simulink model "population_growth"  (R2017b)
settings: Solver=FixedStepDiscrete  StartTime=2010  StopTime=2100  FixedStep=1  MaxStep=1  RelTol=1e-3  EnableMultiTasking=on
PostLoadFcn:
  | load model_parameters
  | % msgbox('Model parameters loaded into base workspace!','Loaded')
values from neighbouring files (symbols this model uses):
  P_2010 = round([P_2010 P_2010].*[male_ratio(1:101) (1-male_ratio(1:101))])    [define_data.m]    (also in model_parameters.mat = [2183279 2225429 2206265 2148270 2142055 2136850 2109005 211)
  p_death_f = ATable(:,5)    [define_data.m]    (also in model_parameters.mat = [0.006096 0.000434 0.000256 0.000192 0.000148 0.000136 0.000)
  p_death_m = ATable(:,2)    [define_data.m]    (also in model_parameters.mat = [0.007379 0.000494 0.000317 0.000241 0.0002 0.000179 0.00016)
  P_immigrants = round(P_immigrants)    [define_data.m]    (also in model_parameters.mat = [0 0 0 0 0 0 0 0 0 0 0 0 ... (240 elements, 120x2)])
  r_birth = [zeros(10,1) ... (first row only)    [define_data.m]    (also in model_parameters.mat = [0 0 0 0 0 0 0 0 0 0 0.4 0.4 ... (120 elements, 120x1)])
libraries: simulink x1
Description:
  | This model predicts the population of the
  | United States as it evolves over the next
  | century. Population for the year 2010 and
  | birth rates were gathered from the US
  | Census Bureau. Immigration rates were
  | derived from DHS, and death rates were
  | provided by the Social Security
  | Administration. These parameters are held
  | fixed and propagated forward.
settings Model: Creator=wcampbel  LastModifiedBy=wcampbel
settings DataIOCC: LimitDataPoints=on  SaveFormat=Array
settings OptimizationCC: ExpressionDepthLimit=2147483647  LifeSpan=inf
settings DebuggingCC: SolverPrmCheckMsg=warning  StateNameClashWarn=warning  SFUnexpectedBacktrackingDiag=warning  SFNoUnconditionalDefaultTransitionDiag=warning  SFExecutionAtInitializationDiag=none
settings HardwareCC: ProdBitPerPointer=32  ProdBitPerSizeT=32  ProdBitPerPtrDiffT=32  ProdLargestAtomicFloat=None  ProdIntDivRoundTo=Undefined  ProdEndianess=Unspecified  ProdWordSize=32  ProdHWDeviceType=32-bit Generic
settings ModelReferenceCC: PropagateSignalLabelsOutOfModel=off
settings CodeAppCC: StateflowObjectComments=on
settings GRTTargetCC: TargetLangStandard=C89/C90 (ANSI)  GeneratePreprocessorConditionals=Disable all  CombineOutputUpdateFcns=off  GRTInterface=on
settings ConfigComp: CovMetricSettings=dw  CovHtmlReporting=on  CovSaveCumulativeToWorkspaceVar=on  CovSaveSingleToWorkspaceVar=on  CovExternalEMLEnable=off

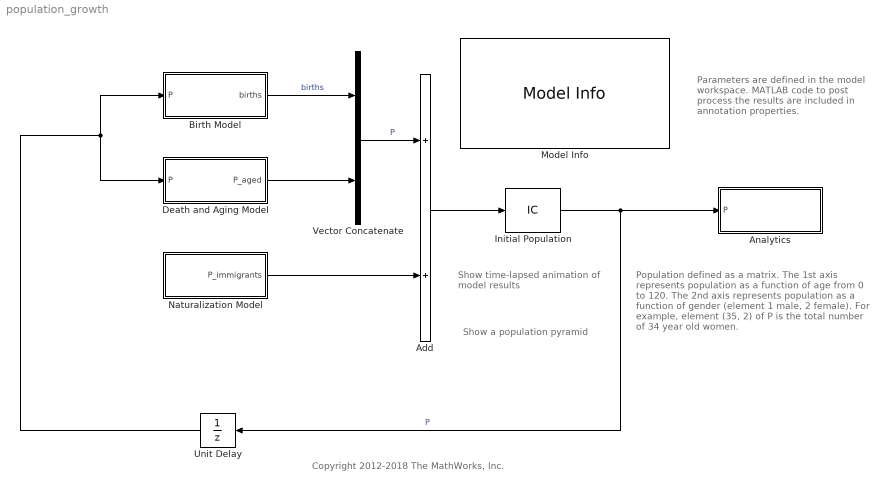
== system population_growth ==
  note: Population defined as a matrix.
      |
      | The 1st axis represents population as
      | a function of age from 0 to 120.
      |
      | The 2nd axis represents population as
      | a function of gender (element 1 male,
      | 2 female).
      |
      | For example, element (35, 2) of P is the
      | total number of 34 year old women.
  note: Parameters are defined in the
      | model workspace. MATLAB code
      | to post process the results are
      | included in annotation properties.
  note: Show a population pyramid
  note: Show time-lapsed animation
      | of model results
  note: Copyright 2012-2018 The MathWorks, Inc.
  Add : Sum
  Analytics : Subsystem
  Birth Model : Subsystem
  Death and Aging Model : Subsystem
  Initial Population : InitialCondition  Priority=3000  Value=P_2010
  Model Info : simulink/Model-Wide Utilities/Model Info  Frame=on  DisplayStringWithTags=%<Description>  HorizontalTextAlignment=Left  LeftAlignmentValue=0.02
  Naturalization Model : Subsystem
  Unit Delay : UnitDelay  SampleTime=-1
  Vector Concatenate : Concatenate  Mode=Multidimensional array
  wires:
  Birth Model/1(births) -> Vector Concatenate/1  "births"
  Death and Aging Model/1(P_aged) -> Vector Concatenate/2
  Naturalization Model/1(P_immigrants) -> Add/2
  Vector Concatenate/1 -> Add/1  "P"
  Add/1 -> Initial Population/1
  Unit Delay/1 -> Birth Model/1(P), Death and Aging Model/1(P)
  Initial Population/1 -> Analytics/1(P), Unit Delay/1  "P"

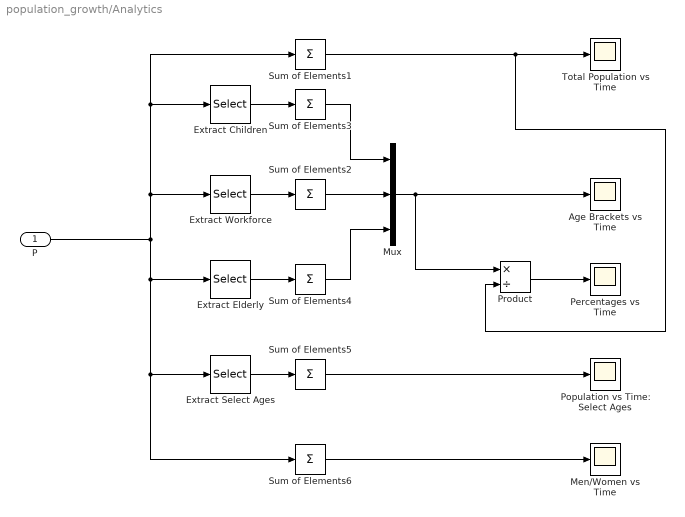
== system population_growth/Analytics ==
  P : Inport
  Age Brackets vs Time : Scope
      settings: Priority=1
  Extract Children : Selector  NumberOfDimensions=2  InputPortWidth=3  IndexOptions=Index vector (dialog),Select all  Indices=[1:18],2  OutputSizes=1,1
  Extract Elderly : Selector  NumberOfDimensions=2  InputPortWidth=3  IndexOptions=Index vector (dialog),Select all  Indices=[67:120],2  OutputSizes=1,1
  Extract Select Ages : Selector  NumberOfDimensions=2  InputPortWidth=3  IndexOptions=Index vector (dialog),Select all  Indices=[1:10:120],2  OutputSizes=1,1
  Extract Workforce : Selector  NumberOfDimensions=2  InputPortWidth=3  IndexOptions=Index vector (dialog),Select all  Indices=[19:66],2  OutputSizes=1,1
  Men/Women vs Time : Scope
      settings: Priority=1
  Mux : Mux  Inputs=3
  Percentages vs Time : Scope
      settings: Priority=1
  Population vs Time: Select Ages : Scope
      settings: Priority=1
  Product : Product  Inputs=*/  RndMeth=Zero
  Sum of Elements{1..4} (4 alike) : Sum  Inputs=+  CollapseDim=2
  Sum of Elements5 : Sum  Inputs=+  CollapseMode=Specified dimension  CollapseDim=2
  Sum of Elements6 : Sum  Inputs=+  CollapseMode=Specified dimension
  Total Population vs Time : Scope
      settings: Priority=1
  wires:
  Sum of Elements1/1 -> Total Population vs Time/1, Product/2
  P/1 -> Sum of Elements1/1, Extract Children/1, Extract Workforce/1, Extract Select Ages/1, Sum of Elements6/1, Extract Elderly/1
  Extract Workforce/1 -> Sum of Elements2/1
  Sum of Elements2/1 -> Mux/2
  Extract Children/1 -> Sum of Elements3/1
  Extract Elderly/1 -> Sum of Elements4/1
  Mux/1 -> Age Brackets vs Time/1, Product/1
  Sum of Elements3/1 -> Mux/1
  Sum of Elements4/1 -> Mux/3
  Product/1 -> Percentages vs Time/1
  Extract Select Ages/1 -> Sum of Elements5/1
  Sum of Elements5/1 -> Population vs Time: Select Ages/1
  Sum of Elements6/1 -> Men/Women vs Time/1

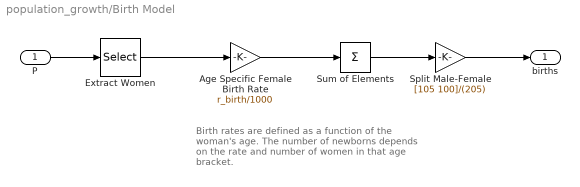
== system population_growth/Birth Model ==
  note: Birth rates are defined as a function
      | of the woman's age. The number of
      | newborns depends on the rate and
      | number of women in that age bracket.
  P : Inport
  Age Specific Female Birth Rate : Gain  Gain=r_birth/1000
  Extract Women : Selector  NumberOfDimensions=2  InputPortWidth=3  IndexOptions=Select all,Index vector (dialog)  Indices=[1 3],2  OutputSizes=1,1
  Split Male-Female : Gain  Gain=[105 100]/(205)
  Sum of Elements : Sum  Inputs=+
  births : Outport
  wires:
  P/1 -> Extract Women/1
  Age Specific Female Birth Rate/1 -> Sum of Elements/1
  Sum of Elements/1 -> Split Male-Female/1
  Extract Women/1 -> Age Specific Female Birth Rate/1
  Split Male-Female/1 -> births/1

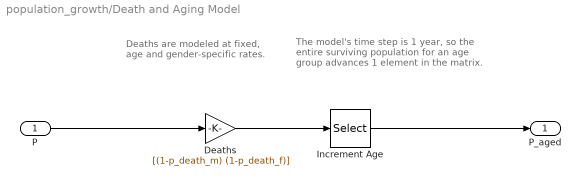
== system population_growth/Death and Aging Model ==
  note: Deaths are modeled
      | at fixed, age and
      | gender-specific rates.
  note: The model's time step is 1 year,
      | so the entire surviving population
      | for an age group advances 1
      | element in the matrix.
  P : Inport
  Deaths : Gain  Gain=[(1-p_death_m) (1-p_death_f)]
  Increment Age : Selector  NumberOfDimensions=2  InputPortWidth=101  IndexOptions=Index vector (dialog),Select all  Indices=[1:119],1  OutputSizes=1,1
  P_aged : Outport
  wires:
  Increment Age/1 -> P_aged/1
  P/1 -> Deaths/1
  Deaths/1 -> Increment Age/1

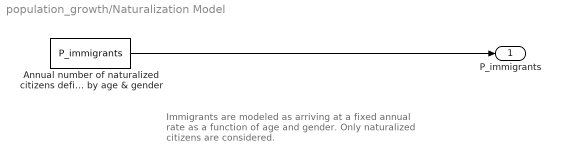
== system population_growth/Naturalization Model ==
  note: Immigrants are modeled as arriving at a
      | fixed annual rate as a function of age and
      | gender. Only naturalized citizens are
      | considered.
  Annual number of naturalized citizens defined by age & gender : Constant  Value=P_immigrants
  P_immigrants : Outport
  wires:
  Annual number of naturalized citizens defined by age & gender/1 -> P_immigrants/1
